simulink model "FILTRO_KALMAN"  (R2017b)
settings: Solver=VariableStepAuto  StartTime=0.0  StopTime=4.25  RelTol=1e-3
undefined symbols (not defined in the file or in its folder): Discrete, Time
libraries: ctrlSharedLib x2
settings Model: Creator=Dr. Candia  LastModifiedBy=Dr. Candia

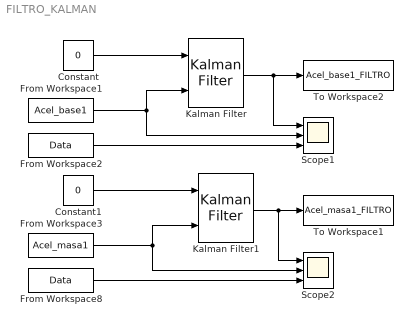
== system FILTRO_KALMAN ==
  Constant : Constant  Value=0
  Constant1 : Constant  Value=0
  From Workspace1 : FromWorkspace  VariableName=Acel_base1  SampleTime=0.01
  From Workspace2 : FromWorkspace  VariableName=Data  SampleTime=0
  From Workspace3 : FromWorkspace  VariableName=Acel_masa1  SampleTime=0.01
  From Workspace8 : FromWorkspace  VariableName=Data  SampleTime=0
  Kalman Filter : ctrlSharedLib/Kalman Filter  TimeDomain=Discrete-Time  UseCurrentEstimator=on  ModelSource=Individual A, B, C, D matrices  ModelSourceVariable=ss(0.95,1,1,0,1)  A=0.95  B=1  C=1  D=0  NumberOfStates=1  NumberOfInputs=1  NumberOfOutputs=1  InitialEstimateSource=Dialog  X0=0  P0=10  UseK=off  UseGH=off  NumberOfProcessNoiseInputs=1  G=1  TimeInvariantG=on  H=0  TimeInvariantH=on  Q=0.05  TimeInvariantQ=on  R=1  TimeInvariantR=on  N=0  TimeInvariantN=on  AddInputPort=on  AddEnablePort=off  OutputEstimatedY=off  OutputP=off  Ts=-1
      settings: SourceProductBaseCode=CT
  Kalman Filter1 : ctrlSharedLib/Kalman Filter  TimeDomain=Discrete-Time  UseCurrentEstimator=on  ModelSource=Individual A, B, C, D matrices  ModelSourceVariable=ss(0.95,1,1,0,1)  A=0.95  B=1  C=1  D=0  NumberOfStates=1  NumberOfInputs=1  NumberOfOutputs=1  InitialEstimateSource=Dialog  X0=0  P0=10  UseK=off  UseGH=off  NumberOfProcessNoiseInputs=1  G=1  TimeInvariantG=on  H=0  TimeInvariantH=on  Q=0.05  TimeInvariantQ=on  R=1  TimeInvariantR=on  N=0  TimeInvariantN=on  AddInputPort=on  AddEnablePort=off  OutputEstimatedY=off  OutputP=off  Ts=-1
      settings: SourceProductBaseCode=CT
  Scope1 : Scope  NumInputPorts=3
  Scope2 : Scope  NumInputPorts=3
  To Workspace1 : ToWorkspace  VariableName=Acel_masa1_FILTRO  SaveFormat=Structure With Time  SampleTime=-1
  To Workspace2 : ToWorkspace  VariableName=Acel_base1_FILTRO  SaveFormat=Structure With Time  SampleTime=-1
  wires:
  From Workspace3/1 -> Kalman Filter1/2, Scope2/2
  From Workspace1/1 -> Kalman Filter/2, Scope1/2
  From Workspace2/1 -> Scope1/3
  Kalman Filter/1 -> To Workspace2/1, Scope1/1
  From Workspace8/1 -> Scope2/3
  Kalman Filter1/1 -> To Workspace1/1, Scope2/1
  Constant/1 -> Kalman Filter/1
  Constant1/1 -> Kalman Filter1/1
